simulink model "TheSteeringFuzzyController"  (R2021a)
settings: Solver=VariableStepAuto  StartTime=0.0  StopTime=10.0  RelTol=1e-3
settings Model: Creator=rasm4  LastModifiedBy=rasm4

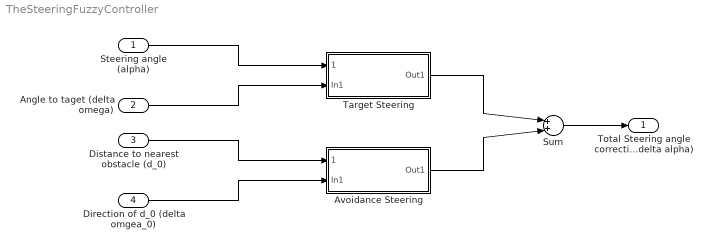
== system TheSteeringFuzzyController ==
  Steering angle (alpha) : Inport
  Angle to taget (delta omega) : Inport  Port=2
  Distance to nearest obstacle (d_0) : Inport  Port=3
  Direction of d_0 (delta omgea_0) : Inport  Port=4
  Avoidance Steering : Subsystem
  Sum : Sum  Inputs=|++|
  Target Steering : Subsystem
  Total Steering angle correction (delta alpha) : Outport
  wires:
  Target Steering/1(Out1) -> Sum/1
  Avoidance Steering/1(Out1) -> Sum/2
  Sum/1 -> Total Steering angle correction (delta alpha)/1
  Steering angle (alpha)/1 -> Target Steering/1
  Angle to taget (delta omega)/1 -> Target Steering/2(In1)
  Distance to nearest obstacle (d_0)/1 -> Avoidance Steering/1
  Direction of d_0 (delta omgea_0)/1 -> Avoidance Steering/2(In1)

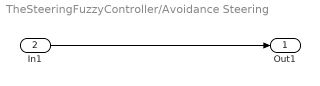
== system TheSteeringFuzzyController/Avoidance Steering ==
  In1 : Inport  Port=2
  Out1 : Outport
  wires:
  In1/1 -> Out1/1

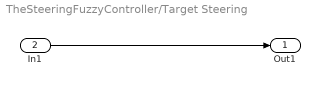
== system TheSteeringFuzzyController/Target Steering ==
  In1 : Inport  Port=2
  Out1 : Outport
  wires:
  In1/1 -> Out1/1
